simulink model "engine_R_2016b"  (R2017a)
settings: Solver=FixedStepDiscrete  StartTime=0.0  StopTime=30.0  FixedStep=0.05  RelTol=1e-3
InitFcn:
  | loadvar
values from neighbouring files (symbols this model uses):
  x0 = [50, 50, 1.14275, 1.53787]    [loadvar.m]
settings Model: Creator=robin  LastModifiedBy=robin

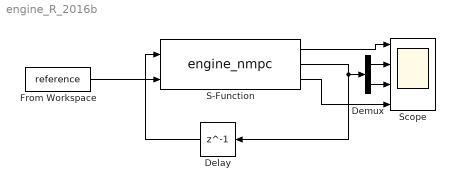
== system engine_R_2016b ==
  Delay : Delay  DelayLength=1  InitialCondition=x0
  Demux : Demux  Outputs=2
  From Workspace : FromWorkspace  VariableName=reference  SampleTime=0
  S-Function : S-Function  FunctionName=engine_nmpc  SFunctionDeploymentMode=off  EnableBusSupport=off
  Scope : Scope  NumInputPorts=4
  wires:
  S-Function/2 -> Demux/1, Delay/1
  Delay/1 -> S-Function/1
  S-Function/1 -> Scope/1
  S-Function/3 -> Scope/4
  Demux/1 -> Scope/2
  Demux/2 -> Scope/3
  From Workspace/1 -> S-Function/2
